simulink model "rom_sim"  (R2013b)
settings: Solver=ode45  StartTime=0.0  StopTime=10.0  RelTol=1e-3
libraries: xbsIndex_r4 x4
settings Model: Creator=root  LastModifiedBy=root

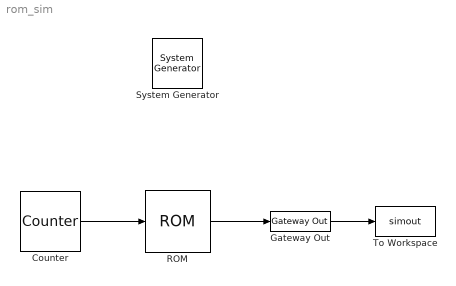
== system rom_sim ==
  " System Generator" : xbsIndex_r4/ System Generator  Tag=genX  xilinxfamily=Kintex7  part=xc7k325t  speed=-3  package=fbg676  synthesis_tool=XST  clock_wrapper=Clock Enables  directory=./netlist  proj_type=Project Navigator  Synth_file=XST Defaults  Impl_file=ISE Defaults  testbench=off  simulink_period=1  sysclk_period=10  dcm_input_clock_period=10  incr_netlist=off  trim_vbits=Everywhere in SubSystem  dbl_ovrd=According to Block Masks  core_generation=According to Block Masks  run_coregen=off  deprecated_control=off  eval_field=0  block_type=sysgen
  Counter : xbsIndex_r4/Counter  cnt_type=Free Running  cnt_to=Inf  operation=Up  start_count=0  cnt_by_val=1  arith_type=Unsigned  n_bits=10  bin_pt=0  load_pin=off  rst=off  en=off  explicit_period=on  period=1  dbl_ovrd=off  use_behavioral_HDL=off  implementation=Fabric  block_type=counter
  Gateway Out : xbsIndex_r4/Gateway Out  inherit_from_input=off  hdl_port=on  timing_constraint=None  locs_specified=off  LOCs={}  UseAsDAC=off  DACChannel='1'  block_type=gatewayout
  ROM : xbsIndex_r4/ROM  depth=1024  initVector="[0.77132    0.020752     0.63365      0.7488     0.49851      0.2248     0.19806     0.76053     0.16911     0.08834     0.68536     0.95339   0.0039483     0.51219     0.81262     0.61253     0.72176     0.29188     0.91777     0.71458     0.54254     0.14217     0.37334     0.67413     0.44183     0.43401     0.61777     0.51314      0.6504     0.60104     0.80522     0.52165     0.90865     0.31924    0.090459      0.3007     0.11398     0.82868    0.046896     0.62629     0.54759     0.81929     0.19895     0.85685     0.35165     0.75465     0.29596     0.88394     0.32551     0.16502     0.39253     0.09346     0.82111     0.15115     0.38411     0.94426     0.98763      0.4563     0.82612     0.25137     0.59737     0.90283     0.53456      0.5902    0.039282     0.35718    0.079613     0.30546     0.33072     0.77383    0.039959     0.42949     0.31493     0.63649     0.34635    0.043097     0.87992     0.76324      0.8781     0.41751     0.60558     0.51347     0.59784     0.26222     0.30087      0.0254     0.30306     0.24208     0.55758     0.56551     0.47513      0.2928    0.064251     0.97882     0.33971     0.49505     0.97708     0.44077     0.31827      0.5198     0.57814     0.85393    0.068097     0.46453     0.78195      0.7186     0.58602    0.037094     0.35066     0.56319     0.29973     0.51233     0.67347     0.15919    0.050478     0.33782     0.10806      0.1789     0.88583     0.36536     0.21877      0.7525     0.10688      0.7446     0.46979     0.59826     0.14762     0.18403     0.64507    0.048628     0.24861     0.54241     0.22677     0.38141     0.92223     0.92536     0.56675     0.53347     0.01486      0.9779     0.57303     0.79176     0.56156     0.87734      0.5842     0.70885     0.14853     0.42845     0.69389     0.10462     0.43961      0.1662     0.50698     0.81904    0.090107     0.80007     0.56513     0.58935      0.1981     0.43612      0.2959    0.037558    0.030685     0.45311     0.74486      0.5573     0.38511     0.16807     0.83826     0.59905     0.78271     0.84851     0.60316     0.78106     0.61574    0.021165     0.75046     0.17604     0.45851     0.51312     0.48402     0.84439     0.17481    0.014635     0.84876     0.74267      0.4567      0.4169     0.11673     0.33868    0.094659     0.71583    0.077085     0.20595     0.57378     0.29383     0.65573     0.80357     0.35121     0.09344     0.81332     0.78487     0.39342     0.86448     0.38403      0.2573      0.8294     0.73638      0.5076     0.64433     0.21319     0.89571     0.96595       0.317     0.86555     0.31028    0.025264    0.049195     0.18463    0.069033     0.25748     0.91358     0.45785     0.13021     0.80989     0.40347    0.024433     0.85683     0.27429     0.70911     0.35577     0.79431     0.84462     0.53815     0.55909     0.12251     0.37764     0.42875     0.51121     0.89176     0.30021     0.39644     0.79327     0.41228     0.18487     0.84025     0.56927     0.06005     0.98892     0.22878      0.6147     0.36803     0.80278     0.62756     0.82122     0.28825      0.2748     0.60105     0.93851      0.7073      0.2634     0.12234     0.45872     0.97481     0.68057     0.19325    0.046739     0.95264     0.85865      0.8279      0.9639     0.59894     0.93092     0.14677     0.11396     0.37203     0.76656     0.32114     0.63804   0.0092211     0.54347     0.33775     0.89802     0.94071     0.38412     0.39612     0.89728    0.058822     0.40538     0.13018    0.086969     0.78396     0.30457     0.58406     0.87847     0.88079     0.60095     0.64523    0.056628     0.29748     0.69177     0.18903     0.80301     0.51476     0.75729     0.17779     0.08262     0.48207     0.52885     0.69631     0.20476     0.67137     0.79327    0.041738     0.96336     0.97539     0.55066    0.064907     0.34524     0.02043     0.80085     0.20793     0.14325     0.69989     0.05795     0.25661     0.51033     0.99526     0.14652     0.44951     0.60144    0.097272     0.28873 ...(+8287 chars)]"  distributed_mem=Block RAM  rst=off  init_reg=0  en=off  latency=1  gui_display_data_type=Fixed-point  arith_type="Signed  (2's comp)"  n_bits=16  bin_pt=14  preci_type=Single  exp_width=8  frac_width=24  dbl_ovrd=off  optimize=Area  use_rpm=on  block_type=sprom
  To Workspace : ToWorkspace  VariableName=simout  SampleTime=-1  SaveFormat=Timeseries
  wires:
  ROM/1 -> Gateway Out/1
  Gateway Out/1 -> To Workspace/1
  Counter/1 -> ROM/1
